simulink model "sl_MCI_sincrono"  (R2016b)
settings: Solver=VariableStepAuto  StartTime=0.0  StopTime=t_sim  RelTol=1e-3
values from neighbouring files (symbols this model uses):
  A = 1    [prueba_persecucionPURA.m]    (also in pruebas_MCI.m = 3; pruebas_modelo.m = 30; tray_parab.m = in(1))
  D = 10    [pruebas_MCI.m]    (also in tray_parab.m = in(2))
  omega_sat = [-0.2618 0.2618]    [prueba_persecucionPURA.m]    (also in pruebas_MCD.m; pruebas_MCI.m = [-0.2618/10 0.2618/10]; pruebas_control.m; pruebas_control_P2.m)
  pos_init = [0;0;0]    [prueba_persecucionPURA.m]    (also in pruebas_MCD.m; pruebas_MCI.m = [0;0;0.2915]; pruebas_control.m; pruebas_control_P2.m)
  tetha_d_sat = [-0.75 0.75]    [prueba_persecucionPURA.m]    (also in pruebas_MCD.m; pruebas_MCI.m = [-0.75/2 0.75/2]; pruebas_control.m; pruebas_control_P2.m)
settings Model: Creator=marrcogrova  LastModifiedBy=Javi Owo

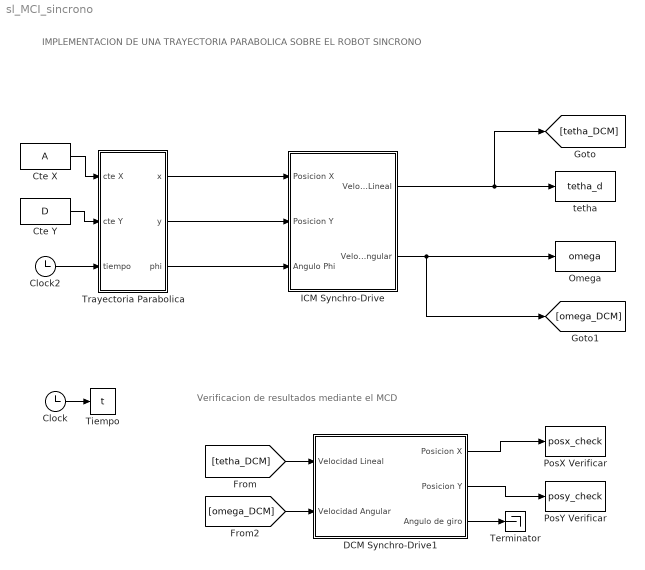
== system sl_MCI_sincrono ==
  note: IMPLEMENTACION DE UNA TRAYECTORIA PARABOLICA
      | SOBRE EL ROBOT SINCRONO
  note: Verificacion de resultados mediante el MCD
  Clock : Clock
  Clock2 : Clock
  Cte X : Constant  Value=A
  Cte Y : Constant  Value=D
  DCM Synchro-Drive1 : Subsystem
  ICM Synchro-Drive : Subsystem
  "Omega " : ToWorkspace  VariableName=omega  SampleTime=-1
  PosX Verificar : ToWorkspace  VariableName=posx_check  SampleTime=-1
  PosY Verificar : ToWorkspace  VariableName=posy_check  SampleTime=-1
  Terminator : Terminator
  Tiempo : ToWorkspace  VariableName=t  SampleTime=-1
  "Trayectoria Parabolica " : Subsystem
  tetha : ToWorkspace  VariableName=tetha_d  SampleTime=-1
  wires:
  Clock/1 -> Tiempo/1
  "Trayectoria Parabolica "/1("x ") -> ICM Synchro-Drive/1(" Posicion X ")
  "Trayectoria Parabolica "/2("y ") -> ICM Synchro-Drive/2(Posicion Y)
  ICM Synchro-Drive/2(Velocidad Angular) -> "Omega "/1, [omega_DCM]
  ICM Synchro-Drive/1(Velocidad Lineal) -> [tetha_DCM], tetha/1
  Cte X/1 -> "Trayectoria Parabolica "/1(cte X)
  DCM Synchro-Drive1/2(Posicion Y) -> PosY Verificar/1
  DCM Synchro-Drive1/1(Posicion X) -> PosX Verificar/1
  "Trayectoria Parabolica "/3("phi ") -> ICM Synchro-Drive/3(Angulo Phi)
  [tetha_DCM] -> DCM Synchro-Drive1/1(Velocidad Lineal)
  [omega_DCM] -> DCM Synchro-Drive1/2(Velocidad Angular)
  DCM Synchro-Drive1/3(Angulo de giro) -> Terminator/1
  Clock2/1 -> "Trayectoria Parabolica "/3(tiempo)
  Cte Y/1 -> "Trayectoria Parabolica "/2("cte Y ")

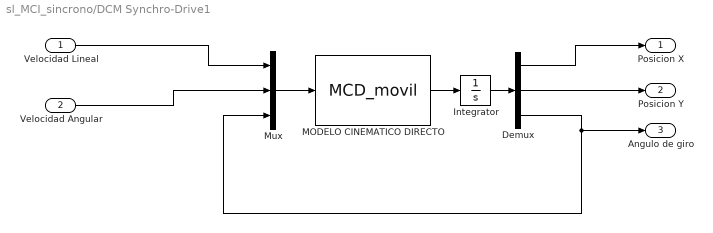
== system sl_MCI_sincrono/DCM Synchro-Drive1 ==
  Velocidad Lineal : Inport
  Velocidad Angular : Inport  Port=2
  Demux : Demux  Outputs=3
  Integrator : Integrator  InitialCondition=pos_init
  MODELO CINEMATICO DIRECTO : MATLABFcn  MATLABFcn=MCD_movil  OutputDimensions=3
  Mux : Mux  Inputs=3
  Posicion X : Outport
  Posicion Y : Outport  Port=2
  Angulo de giro : Outport  Port=3
  wires:
  Integrator/1 -> Demux/1
  Demux/3 -> Angulo de giro/1, Mux/3
  Demux/1 -> Posicion X/1
  Demux/2 -> Posicion Y/1
  Mux/1 -> MODELO CINEMATICO DIRECTO/1
  MODELO CINEMATICO DIRECTO/1 -> Integrator/1
  Velocidad Lineal/1 -> Mux/1
  Velocidad Angular/1 -> Mux/2

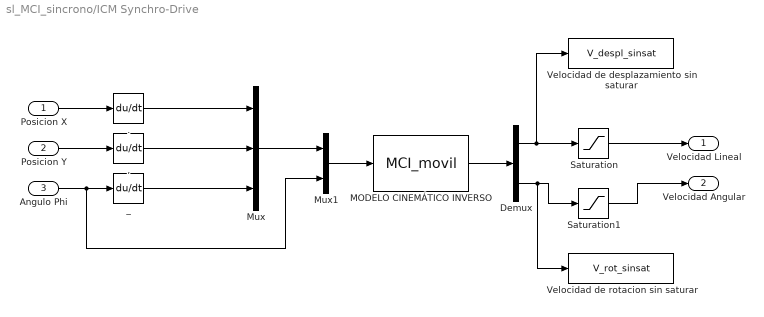
== system sl_MCI_sincrono/ICM Synchro-Drive ==
  " Posicion X " : Inport
  Posicion Y : Inport  Port=2
  Angulo Phi : Inport  Port=3
  , : Derivative
  . : Derivative
  Demux : Demux  Outputs=2
  MODELO CINEMÁTICO INVERSO : MATLABFcn  MATLABFcn=MCI_movil  OutputDimensions=2
  Mux : Mux  Inputs=3
  Mux1 : Mux  Inputs=2
  Saturation : Saturate  UpperLimit=tetha_d_sat(2)  LowerLimit=tetha_d_sat(1)  ZeroCross=off
  Saturation1 : Saturate  UpperLimit=omega_sat(2)  LowerLimit=omega_sat(1)  ZeroCross=off
  Velocidad de desplazamiento sin saturar : ToWorkspace  VariableName=V_despl_sinsat  SampleTime=-1
  Velocidad de rotacion sin saturar : ToWorkspace  VariableName=V_rot_sinsat  SampleTime=-1
  _ : Derivative
  Velocidad Lineal : Outport
  Velocidad Angular : Outport  Port=2
  wires:
  MODELO CINEMÁTICO INVERSO/1 -> Demux/1
  Mux/1 -> Mux1/1
  Angulo Phi/1 -> Mux1/2, _/1
  Saturation1/1 -> Velocidad Angular/1
  Saturation/1 -> Velocidad Lineal/1
  " Posicion X "/1 -> ./1
  ./1 -> Mux/1
  Posicion Y/1 -> ,/1
  ,/1 -> Mux/2
  _/1 -> Mux/3
  Demux/2 -> Velocidad de rotacion sin saturar/1, Saturation1/1
  Demux/1 -> Velocidad de desplazamiento sin saturar/1, Saturation/1
  Mux1/1 -> MODELO CINEMÁTICO INVERSO/1

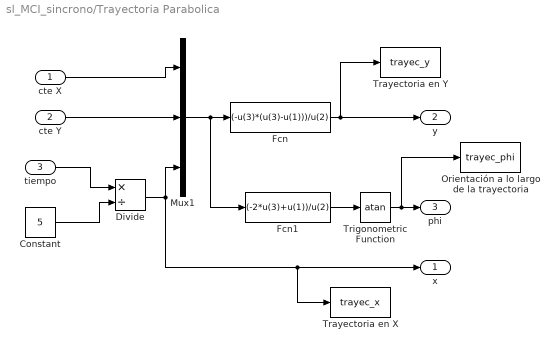
== system sl_MCI_sincrono/Trayectoria Parabolica  ==
  cte X : Inport
  "cte Y " : Inport  Port=2
  tiempo : Inport  Port=3
  Constant : Constant  Value=5
  Divide : Product  Inputs=*/
  Fcn : Fcn  Expr=(-u(3)*(u(3)-u(1)))/u(2)
  Fcn1 : Fcn  Expr=(-2*u(3)+u(1))/u(2)
  Mux1 : Mux  Inputs=3
  Orientación a lo largo de la trayectoria : ToWorkspace  VariableName=trayec_phi  SampleTime=-1
  Trayectoria en X : ToWorkspace  VariableName=trayec_x  SampleTime=-1
  Trayectoria en Y : ToWorkspace  VariableName=trayec_y  SampleTime=-1
  Trigonometric Function : Trigonometry  Operator=atan  OutputSignalType=real
  "x " : Outport
  "y " : Outport  Port=2
  "phi " : Outport  Port=3
  wires:
  Fcn/1 -> Trayectoria en Y/1, "y "/1
  cte X/1 -> Mux1/1
  Mux1/1 -> Fcn/1, Fcn1/1
  Fcn1/1 -> Trigonometric Function/1
  Trigonometric Function/1 -> Orientación a lo largo de la trayectoria/1, "phi "/1
  Constant/1 -> Divide/2
  Divide/1 -> Trayectoria en X/1, "x "/1, Mux1/3
  tiempo/1 -> Divide/1
  "cte Y "/1 -> Mux1/2
